simulink model "Cart_Pendulum_Non_Linear"  (R2019b)
settings: Solver=VariableStepAuto  StartTime=0.0  StopTime=10.0  RelTol=1e-3
values from neighbouring files (symbols this model uses):
  Model_Constants = [Mc , m , lm , gm]    [Main.m]
  x0_a = [0.2 , (20*pi)/180 , 0 , 0]'    [Main.m]
  x0_b = [0 pi 0 0]    [Main.m]
undefined symbols (not defined in the file or in its folder): K
settings Model: Creator=don  LastModifiedBy=don

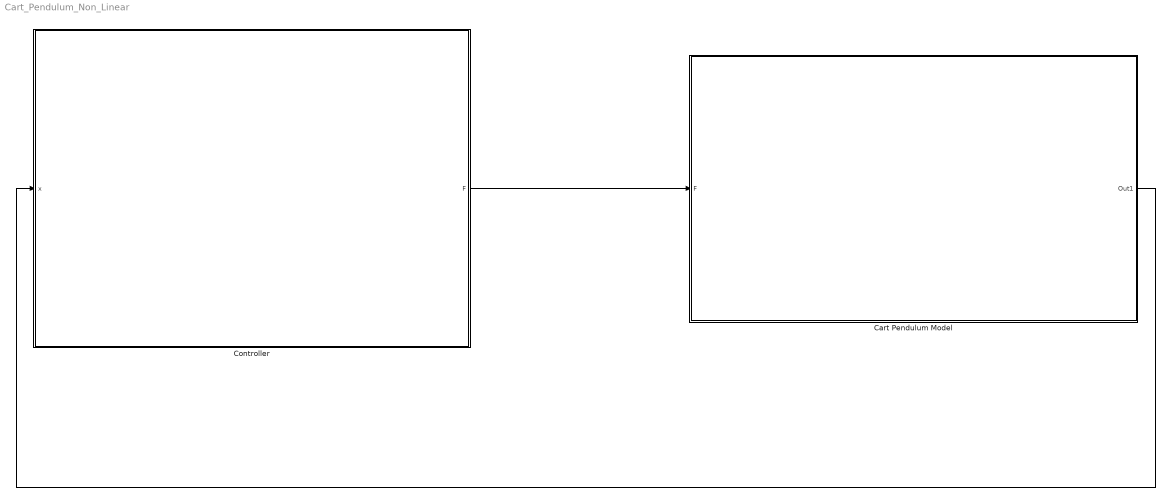
== system Cart_Pendulum_Non_Linear ==
  Cart Pendulum Model : Subsystem
  Controller : Subsystem
  wires:
  Controller/1(F) -> Cart Pendulum Model/1(F)
  Cart Pendulum Model/1(Out1) -> Controller/1(x)

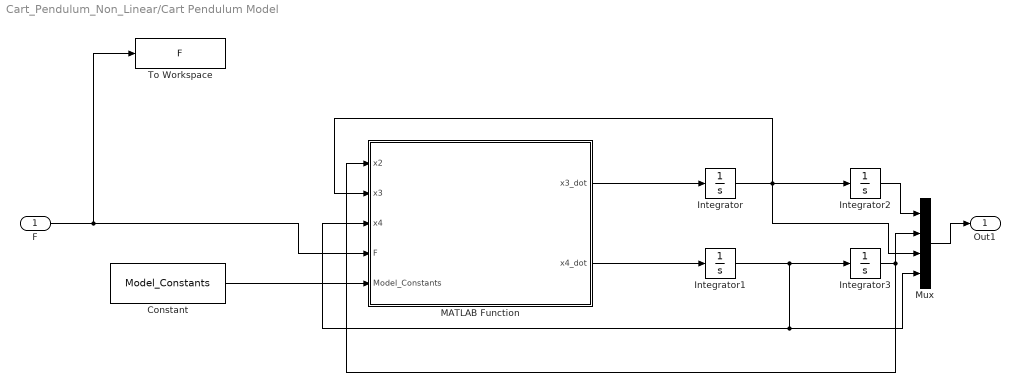
== system Cart_Pendulum_Non_Linear/Cart Pendulum Model ==
  F : Inport
  Constant : Constant  Value=Model_Constants
  Integrator : Integrator  InitialCondition=x0_a
  Integrator1 : Integrator  InitialCondition=x0_b
  Integrator2 : Integrator
  Integrator3 : Integrator
  MATLAB Function : MATLAB Function  TreatAsAtomicUnit=on
  Mux : Mux
  To Workspace : ToWorkspace  VariableName=F  SaveFormat=Timeseries  SampleTime=-1
  Out1 : Outport
  wires:
  MATLAB Function/1(x3_dot) -> Integrator/1
  MATLAB Function/2(x4_dot) -> Integrator1/1
  F/1 -> To Workspace/1, MATLAB Function/4(F)
  Constant/1 -> MATLAB Function/5(Model_Constants)
  Integrator/1 -> Mux/3, MATLAB Function/2(x3), Integrator2/1
  Integrator2/1 -> Mux/1
  Integrator3/1 -> MATLAB Function/1(x2), Mux/2
  Mux/1 -> Out1/1
  Integrator1/1 -> MATLAB Function/3(x4), Mux/4, Integrator3/1

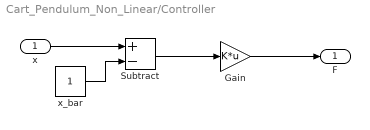
== system Cart_Pendulum_Non_Linear/Controller ==
  x : Inport
  Gain : Gain  Gain=K*u
  Subtract : Sum  Inputs=+-
  x_bar : Constant
  F : Outport
  wires:
  x/1 -> Subtract/1
  Subtract/1 -> Gain/1
  Gain/1 -> F/1
  x_bar/1 -> Subtract/2

== matlab function Cart_Pendulum_Non_Linear/Cart Pendulum Model/MATLAB Function ==
  data: x2 input; x3_dot output; x3 input; x4 input; F input; Model_Constants input; x4_dot output
function [x3_dot, x4_dot] = NonLinearEquations(x2 , x3 , x4 , F , Model_Constants  )
    
    % Model Constants
    Mc = Model_Constants(1);
    m  = Model_Constants(2);
    lm = Model_Constants(3);
    gm = Model_Constants(4);

    % Equations for x3 dot: and x4 dot:
    x3_nancy  = (x4^2)*lm*sin(x2) - gm*sin(x2) * cos(x2) + F;
    x3_donkey = Mc + m - m*cos(x2)*cos(x2);
    x3_dot = x3_nancy / x3_donkey;
    
    x4_nancy  = -lm*sin(x2)*cos(x2)*(x4^2) + gm*(Mc + m)*sin(x2) - cos(x2)*F;
    x4_donkey = l*(Mc  + m - m*cos(x2)*cos(x2) );
    x4_dot = x4_nancy / x4_donkey;


end
